simulink model "controller_r12"  (Simulink 4.00)
settings: Solver=ode45  StartTime=0.0  StopTime=1.0  RelTol=1e-3
undefined symbols (not defined in the file or in its folder): Imax, Imin, KController, KCurrent, KPreset, Kt, TiController, TiCurrent
settings Model: LastModifiedBy=ESI ITI GmbH  LimitDataPoints=off  ExtModeTrigMode=oneshot  ExtModeArmWhenConnect=off

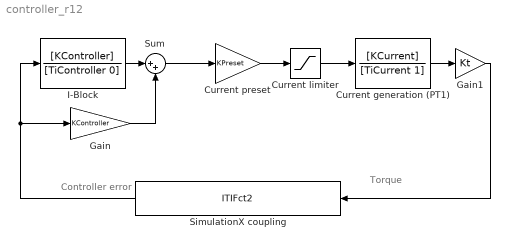
== system controller_r12 ==
  note: Controller
      | error
  note: Torque
  Current limiter : Saturate  UpperLimit=Imax  LowerLimit=Imin  LinearizeAsGain=on
  Current preset : Gain  Gain=KPreset  Multiplication=Element-wise(K.*u)  SaturateOnIntegerOverflow=on
  Current generation (PT1) : TransferFcn  Numerator=[KCurrent]  Denominator=[TiCurrent 1]  AbsoluteTolerance=auto  Realization=auto
  Gain : Gain  Gain=KController  Multiplication=Element-wise(K.*u)  SaturateOnIntegerOverflow=on
  Gain1 : Gain  Gain=Kt  Multiplication=Element-wise(K.*u)  SaturateOnIntegerOverflow=on
  I-Block : TransferFcn  Numerator=[KController]  Denominator=[TiController 0]  AbsoluteTolerance=auto  Realization=auto
  SimulationX coupling : S-Function  Orientation=left  FunctionName=ITIFct2  PortCounts=[]  SFunctionModules=''  Parameters=ip, port, ts, nIn, nOut  mask{ip='localhost', port=4097, ts=0.001, nIn=1, nOut=1}
      mask prompts: ip "Address: ip"; port "Port Number: port [-]"; ts "Communication Step Size: ts [s]"; nIn "Input Vector Dimension (to SimulationX): nIn [-]"; nOut "Output Vector Dimension (from SimulationX): nOut [-]"
      mask help: Coupling Element
  Sum : Sum  Inputs=|++  SaturateOnIntegerOverflow=on
  wires:
  I-Block/1 -> Sum/1
  Gain/1 -> Sum/2
  Sum/1 -> Current preset/1
  Current preset/1 -> Current limiter/1
  Current limiter/1 -> Current generation (PT1)/1
  Current generation (PT1)/1 -> Gain1/1
  Gain1/1 -> SimulationX coupling/1
  SimulationX coupling/1 -> I-Block/1, Gain/1
